simulink model "Stateflow_test"  (R2021a)
settings: Solver=FixedStepDiscrete  StartTime=0.0  StopTime=1000000  FixedStep=0.1  RelTol=1e-3
settings Model: EnablePacing=on  Creator=20201588  LastModifiedBy=20201588
settings DataIOCC: ExternalInput=k  SaveOutput=off  SignalLogging=off  DSMLogging=off  SaveTime=off  ReturnWorkspaceOutputs=off

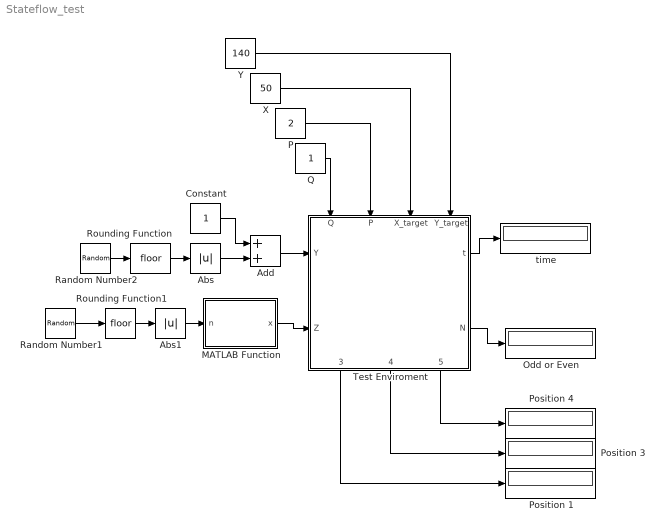
== system Stateflow_test ==
  Abs : Abs
  Abs1 : Abs
  Add : Sum
  Constant : Constant
  MATLAB Function : MATLAB Function  TreatAsAtomicUnit=on
  Odd or Even : Display
  P : Constant  Value=2
  Position 1 : Display
  Position 3 : Display
  Position 4 : Display
  Q : Constant
  Random Number1 : RandomNumber  Variance=100000  SampleTime=0.1
  Random Number2 : RandomNumber  Variance=100000  SampleTime=0.1
  Rounding Function : Rounding
  Rounding Function1 : Rounding
  Test Enviroment : Stateflow chart  TreatAsAtomicUnit=on
      settings: PortSchema="{\"entries\":[{\"content\":{\"sides\":[{\"content\":{\"connectorIds\":[\"In1\",\"In2\"]},\"type\":\"ConnectorPlacement.EquallySpacedRectSide\",\"uuid\":\"30c27bf2-aba7-402c-b200-cd809c499820\"},{\"content\":{\"connectorIds\":[\"Out1\",\"Out2\"],\"side\":\"RIGHT\"},\"type\":\"ConnectorPlacement.EquallySpacedRectSide\",\"uuid\":\"5fb1c3a1-970d-4595-8858-19f50385e32e\"},{\"content\":{\"connectorIds\":[\"In4\",\"In3\",\"In5\",\"In6\"],\"side\":\"TOP\"},\"type\":\"ConnectorPlacement.EquallySpacedRectSide\",\"uuid\":\"36195fad-53c8-499a-9c43-961bfbaf41e7\"},{\"content\":{\"connectorIds\":[\"Out3\",\"Out4\",\"Out5\"],\"side\":\"BOTTOM\"},\"type\":\"ConnectorPlacement.EquallySpacedRectSide\",\"uuid\":\"809a5c53-c969-4d66-b175-34124aee756d\"}]},\"type\":\"ConnectorPlacement.EquallySpacedConnector\",\"uuid\":\"2a5091d1-cc93-467a-a765-baae29c7acb5\"}],\"packageUris\":[\"http://schema.mathworks.com/mf0/Connector/R2020b\"],\"version\":\"1.0\"}"
  X : Constant  Value=50
  Y : Constant  Value=140
  time : Display
  wires:
  Test Enviroment/2(N) -> Odd or Even/1
  Random Number2/1 -> Rounding Function/1
  Test Enviroment/1(t) -> time/1
  Rounding Function/1 -> Abs/1
  MATLAB Function/1(x) -> Test Enviroment/2(Z)
  Rounding Function1/1 -> Abs1/1
  Abs1/1 -> MATLAB Function/1(n)
  Random Number1/1 -> Rounding Function1/1
  Abs/1 -> Add/2
  Add/1 -> Test Enviroment/1(Y)
  Constant/1 -> Add/1
  P/1 -> Test Enviroment/3(P)
  Q/1 -> Test Enviroment/4(Q)
  X/1 -> Test Enviroment/5(X_target)
  Y/1 -> Test Enviroment/6(Y_target)
  Test Enviroment/5(R_rad_target) -> Position 4/1
  Test Enviroment/4(X_rad_target) -> Position 3/1
  Test Enviroment/3(Z_rad_target) -> Position 1/1

== matlab function Stateflow_test/MATLAB Function ==
  data: n input; x output
function x = fcn(n)

r = randi([-10*n 10*n],n,n);

s = randi([1 n],1,1);
f = randi([1 n],1,1);

x = r(s,f);

== stateflow chart Stateflow_test/Test Enviroment ==
  state Odd_or_Even [parallel]
    settings: executionOrder=1
    state Sum_is_odd
      entry:
      X = 1; N = 0;
      during:
      X = rand(Y)+Z;
    state Sum_is_even
      entry:
      X = 2; N = 1;
      during:
      X = rand(Y)+Z;
    (default) -> Sum_is_odd
    Sum_is_odd -> Sum_is_even : [rem(X,2)==0]
    Sum_is_even -> Sum_is_odd : [rem(X,2)==1]
  state Time [parallel]
    settings: executionOrder=2
    state Time_1
      entry, during:
      p = rand(Y);
      t = elapsed(sec);
    state Time_2 [commented out]
      entry, during:
      T = elapsed(sec);
    (default) -> Time_1
    Time_2 -> Time_1 [commented out] : after(1,sec)
    Time_1 -> Time_2 [commented out] : after(1,sec)
  state Position_Example [parallel] [commented out]
    state Block_1 [parallel] [commented out]
      state Pick_Up_Block_1 [commented out]
        en, du:
        P1 =  0;
        exit:
        Pi_1 = 4;
      state Position_Block_1 [commented out]
        du, en:
        P1 = 5*elapsed(sec) + Pi_1;
      state Start [commented out]
        du,en:
        Pi_1 = 0;
      Position_Example.Block_1.Start -> Position_Block_1 [commented out]
      (default) -> Position_Example.Block_1.Start [commented out]
      Pick_Up_Block_1 -> Position_Block_1 [commented out] : [P == 0 & Q ==1 ]
      Position_Block_1 -> Pick_Up_Block_1 [commented out] : [P == 1 & Q == 1]
    state Block_2 [parallel] [commented out]
      state Pick_Up_Block_2 [commented out]
        en, du:
        P2 = 0;
        exit:
        Pi_2 = 4;
      state Position_Block_2 [commented out]
        du, en:
        P2 = 5*elapsed(sec) + Pi_2;
      state Start [commented out]
        du,en:
        Pi_2 = 0;
      Pick_Up_Block_2 -> Position_Block_2 [commented out] : [P == 0 & Q ==2 ]
      Position_Block_2 -> Pick_Up_Block_2 [commented out] : [P == 1 & Q == 2]
      Position_Example.Block_2.Start -> Position_Block_2 [commented out]
      (default) -> Position_Example.Block_2.Start [commented out]
  state Read_Table [parallel]
    settings: executionOrder=3
    state Lookup_Table
      en:
      X_start  =  -228;
      Y_start  = 79;
      [Red_X, Red_Z,  Red_R, ...
      Yel_X, Yel_Z, Yel_R, ...
      Tra_X, Tra_Z, Tra_R, step]  = Lookup;
    state Detecting_Stage
      %This is where the detection
      %of the block would happen
    state Moving_Stage_Yellow
      en,du:
      X_index = (X_target-X_start)/step;
      Y_index = (Y_target-Y_start)/step;
      X_rad_target = interp2(Yel_X,Y_index,X_index);
      R_rad_target = interp2(Yel_R,Y_index,X_index);
      Z_rad_target = interp2(Yel_Z,Y_index,X_index);
    state Moving_Stage_Red
      en,du:
      X_index = (X_target-X_start)/step;
      Y_index = (Y_target-Y_start)/step;
      X_rad_target = interp2(Red_X,Y_index,X_index);
      R_rad_target = interp2(Red_R,Y_index,X_index);
      Z_rad_target = interp2(Red_Z,Y_index,X_index);
    state Transport_Stage
      en,du:
      X_index = (X_target-X_start)/step;
      Y_index = (Y_target-Y_start)/step;
      X_rad_target = interp2(Tra_X,Y_index,X_index);
      R_rad_target = interp2(Tra_R,Y_index,X_index);
      Z_rad_target = interp2(Tra_Z,Y_index,X_index);
    (default) -> Lookup_Table
    Lookup_Table -> Detecting_Stage
    Detecting_Stage -> Moving_Stage_Yellow [order 2] : [Q == 2 & P ==1]
    Detecting_Stage -> Moving_Stage_Red [order 1] : [Q == 1 & P ==1]
    Moving_Stage_Red -> Transport_Stage : [P == 2]
    Moving_Stage_Yellow -> Transport_Stage : [P == 2]
  data: n function_input; x function_output; P1 function_output; P2 function_output; P3 function_output; P4 function_output; P5 function_output; P6 function_output; P7 function_output; P8 function_output; P9 function_output; step_size function_output; Y input; Z input; X local; t output; N output; p local; P input; Q input; Pi_2 local; Pi_1 local; Red_R local; Red_Z local; Red_X local; Tra_X local; Yel_R local; Yel_X local; Yel_Z local; Tra_Z local; step local; Y_start local; X_start local; Z_rad_target output; X_rad_target output; R_rad_target output; X_target input; Y_target input; Tra_R local; X_index local; Y_index local
  function x = rand(n):
    | function x = rand(n)
    |  
    | r = randi([-10*n 10*n],n,n);
    | 
    | s = randi([1 n],1,1);
    | f = randi([1 n],1,1);
    | 
    | x = r(s,f);
  function [P1, P2, P3, P4, P5,  P6,  P7,  P8,  P9, step_size]= Lookup:
    | function [P1, P2, P3, P4, P5,  P6,  P7,  P8,  P9, step_size]= Lookup
    | 
    | step_size = 20
    | 
    | P1 = ...
    |   [0.078490748900463925 0 0 0 0 0 0;
    |    -0.14160324448913111 -0.049572307843604724 0.12708300072520992 0 0 0 ...
    |    0;
    |    -0.27157787377661163 -0.20182258283986637 -0.10634227096077699 0.048525204061919937 ...
    |    0 0 0;
    |    -0.37215450602130229 -0.30994030328141381 -0.23070086145651506 -0.12513068019242732 ...
    |    0.044207338161135111 0 0;
    |    -0.45597476566310996 -0.39644723094061213 -0.32358159546482551 -0.23266896174672444 ...
    |    -0.11132586814638003 0.10678216745830364 0;
    |    -0.52822091878882982 -0.46869829447830874 -0.39813136114620756 -0.3135156344249258 ...
    |    -0.20797697259670342 -0.061121896669658671 0;
    |    -0.59138527368032068 -0.52990747874252764 -0.45929417119146188 -0.37726504619144469 ...
    |    -0.27901154079820384 -0.15302076809051285 0.0499859200990351;
    |    -0.64643227421234584 -0.58139905329097474 -0.5091959536765388 -0.42771137003577658 ...
    |    -0.33297424363263062 -0.21676008945412273 -0.054434792366532522;
    |    -0.62328641003273344 -0.54856621140117323 -0.46648547704422505 -0.3732914885966841 ...
    |    -0.26219124059014348 -0.1162498375777507 0;
    |    -0.65477765533194343 -0.57731612637156482 -0.49417897981862507 -0.40149598471752612 ...
    |    -0.29308567320354412 -0.15527223637806487 0;
    |    -0.67454045864903067 -0.59493539199982293 -0.510868815105908 -0.41825451853521306 ...
    |    -0.31113343840230134 -0.17725387432785519 0;
    |    -0.6008842036628036 -0.51645247029269337 -0.42382031113568408 -0.3170789405401413 ...
    |    -0.18438303533059774 0 0;
    |    -0.67454045864903067 -0.59493539199982293 -0.510868815105908 -0.41825451853521306 ...
    |    -0.31113343840230134 -0.17725387432785519 0;
    |    -0.65477765533194343 -0.57731612637156482 -0.49417897981862507 -0.40149598471752612 ...
    |    -0.29308567320354412 -0.15527223637806487 0;
    |    -0.62328641003273344 -0.54856621140117323 -0.46648547704422505 -0.3732914885966841 ...
    |    -0.26219124059014348 -0.1162498375777507 0;
    |    -0.64643227421234584 -0.58139905329097474 -0.5091959536765388 -0.42771137003577658 ...
    |    -0.33297424363263062 -0.21676008945412273 -0.054434792366532522;
    |    -0.59138527368032068 -0.52990747874252764 -0.45929417119146188 -0.37726504619144469 ...
    |    -0.27901154079820384 -0.15302076809051285 0.0499859200990351;
    |    -0.52822091878882982 -0.46869829447830874 -0.39813136114620756 -0.3135156344249258 ...
    |    -0.20797697259670342 -0.061121896669658671 0;
    |    -0.45597476566310996 -0.39644723094061213 -0.32358159546482551 -0.23266896174672444 ...
    |    -0.11132586814638003 0.10678216745830364 0;
    |    -0.37215450602130229 -0.30994030328141381 -0.23070086145651506 -0.12513068019242732 ...
    |    0.044207338161135111 0 0;
    |    -0.27157787377661163 -0.20182258283986637 -0.10634227096077699 0.048525204061919937 ...
    |    0 0 0;
    |    -0.14160324448913111 -0.049572307843604724 0.12708300072520992 0 0 0 ...
    |    0;
    |    0.078490748900463925 0 0 0 0 0 0];
    | P2 = ...
    |   [-0.12914851440826922 0 0 0 0 0 0;
    |    -0.031147893091569411 -0.077606350910947919 -0.14238184107600749 0 0 ...
    |    0 0;
    |    0.038115006213386052 0.00097753000030033452 -0.049502944336502347 -0.11903370925601538 ...
    |    0 0 0;
    |    0.088172973459990187 0.057915795871910543 0.016451058436103165 -0.039786051111986041 ...
    |    -0.11746414751217649 0 0;
    |    0.12320986517913864 0.099126747790600628 0.064776879140110641 0.017502499912164002 ...
    |    -0.046941591530162037 -0.13735685373267448 0;
    |    0.1455634435709153 0.12775542375045904 0.099864536107933291 0.059724492124420374 ...
    |    0.0042794148117395675 -0.072074838684885761 0;
    |    0.15698816571742835 0.14597603798865905 0.12441834465360993 0.090523742090328235 ...
    |    0.042001398835270945 -0.02510904800516426 -0.11955852667623298;
    |    0.15935403780028756 0.15576457968830729 0.14053907023566314 0.11231467916400005 ...
    |    0.069434622529717827 0.0089891923775578877 -0.075290820322378632;
    |    0.15929172088395394 0.15016609924800148 0.12698191064896727 0.0886980038252953 ...
    |    0.033179981423454109 -0.044399102796648091 0;
    |    0.15903111902237949 0.15519807407823663 0.13611481885448781 0.10132963703365482 ...
    |    0.049298666564871779 -0.023914081850700819 0;
    |    0.15751883351380158 0.15736682441418084 0.14100746879651566 0.10844319967004758 ...
    |    0.058520174583554761 -0.012192524522075769 0;
    |    0.1579339306852009 0.14253431690789742 0.11073471576986624 0.061519876623784726 ...
    |    -0.0083753026802587047 0 0;
    |    0.15751883351380158 0.15736682441418084 0.14100746879651566 0.10844319967004758 ...
    |    0.058520174583554761 -0.012192524522075769 0;
    |    0.15903111902237949 0.15519807407823663 0.13611481885448781 0.10132963703365482 ...
    |    0.049298666564871779 -0.023914081850700819 0;
    |    0.15929172088395394 0.15016609924800148 0.12698191064896727 0.0886980038252953 ...
    |    0.033179981423454109 -0.044399102796648091 0;
    |    0.15935403780028756 0.15576457968830729 0.14053907023566314 0.11231467916400005 ...
    |    0.069434622529717827 0.0089891923775578877 -0.075290820322378632;
    |    0.15698816571742835 0.14597603798865905 0.12441834465360993 0.090523742090328235 ...
    |    0.042001398835270945 -0.02510904800516426 -0.11955852667623298;
    |    0.1455634435709153 0.12775542375045904 0.099864536107933291 0.059724492124420374 ...
    |    0.0042794148117395675 -0.072074838684885761 0;
    |    0.12320986517913864 0.099126747790600628 0.064776879140110641 0.017502499912164002 ...
    |    -0.046941591530162037 -0.13735685373267448 0;
    |    0.088172973459990187 0.057915795871910543 0.016451058436103165 -0.039786051111986041 ...
    |    -0.11746414751217649 0 0;
    |    0.038115006213386052 0.00097753000030033452 -0.049502944336502347 -0.11903370925601538 ...
    |    0 0 0;
    |    -0.031147893091569411 -0.077606350910947919 -0.14238184107600749 0 0 ...
    |    0 0;
    |    -0.12914851440826922 0 0 0 0 0 0];
    | P3 = ...
    |   [-1.1555280696863055 0 0 0 0 0 0;
    |    -1.1192205659593462 -1.0414792570758407 -0.97020857536930272 0 0 0 0 ...
    |    ;
    |    -1.076523722378983 -0.99442110620371293 -0.92022194958143655 -0.85354174926493276 ...
    |    0 0 0;
    |    -1.025793907189114 -0.939403607044929 -0.86268498768041613 -0.79486160328000632 ...
    |    -0.73499578368810314 0 0;
    |    -0.9648803301212161 -0.87465454274782362 -0.7962280648859561 -0.72822149452105855 ...
    |    -0.66920466660723954 -0.617844488214677 0;
    |    -0.89099469902914064 -0.79805571523150021 -0.71934652850130743 -0.65261016858449106 ...
    |    -0.59578454762305888 -0.5471108502163885 0;
    |    -0.80062541277456556 -0.70721682979106137 -0.63053013816735171 -0.5671412488145694 ...
    |    -0.51426512799322155 -0.46972040884091021 -0.43182315125830661;
    |    -0.68964667050168171 -0.59974374696942356 -0.52852816890339194 -0.4712616750560702 ...
    |    -0.42449711714228811 -0.38574650382157327 -0.35320392615379503;
    |    -0.4738513364947603 -0.412793289970719 -0.36503799768109646 -0.32682665292994068 ...
    |    -0.29564281653907476 -0.26975807296212945 0;
    |    -0.32942303811214763 -0.28407437825928533 -0.2494696508978248 -0.22225530228522308 ...
    |    -0.20032238076082171 -0.18228559876685382 0;
    |    -0.16930377815578745 -0.14496139639150155 -0.12670608739343886 -0.11251710743602975 ...
    |    -0.10117618903756062 -0.09190625132479012 0;
    |    0 0 0 0 0 0 0;
    |    0.16930377815578745 0.14496139639150155 0.12670608739343886 0.11251710743602975 ...
    |    0.10117618903756062 0.09190625132479012 0;
    |    0.32942303811214763 0.28407437825928533 0.2494696508978248 0.22225530228522308 ...
    |    0.20032238076082171 0.18228559876685382 0;
    |    0.4738513364947603 0.412793289970719 0.36503799768109646 0.32682665292994068 ...
    |    0.29564281653907476 0.26975807296212945 0;
    |    0.68964667050168171 0.59974374696942356 0.52852816890339194 0.4712616750560702 ...
    |    0.42449711714228811 0.38574650382157327 0.35320392615379503;
    |    0.80062541277456556 0.70721682979106137 0.63053013816735171 0.5671412488145694 ...
    |    0.51426512799322155 0.46972040884091021 0.43182315125830661;
    |    0.89099469902914064 0.79805571523150021 0.71934652850130743 0.65261016858449106 ...
    |    0.59578454762305888 0.5471108502163885 0;
    |    0.9648803301212161 0.87465454274782362 0.7962280648859561 0.72822149452105855 ...
    |    0.66920466660723954 0.617844488214677 0;
    |    1.025793907189114 0.939403607044929 0.86268498768041613 0.79486160328000632 ...
    |    0.73499578368810314 0 0;
    |    1.076523722378983 0.99442110620371293 0.92022194958143655 0.85354174926493276 ...
    |    0 0 0;
    |    1.1192205659593462 1.0414792570758407 0.97020857536930272 0 0 0 0;
    |    1.1555280696863055 0 0 0 0 0 0];
    | P4 = ...
    |   [-0.11480438890444414 -0.0087043704871341727 0 0 0 0 0;
    |    -0.27129154221375518 -0.19669467676343674 -0.093513525421083779 0.084162799376508335 ...
    |    0 0 0;
    |    -0.38979410217880406 -0.32466498232115132 -0.24156701330429597 -0.13095572032037739 ...
    |    0.044976045332462418 0 0;
    |    -0.48861664005099803 -0.42686197626553057 -0.35124331883001292 -0.25724872369268215 ...
    |    -0.13345504395339669 0.072723448912593427 0;
    |    -0.57476980602955541 -0.51324504399375992 -0.44023460899805017 -0.35307531411572796 ...
    |    -0.24569010559136686 -0.10162396951576309 0;
    |    -0.65167507358591581 -0.58813506580271135 -0.51496283941836685 -0.43035746187103235 ...
    |    -0.33028026714588782 -0.20548593687598274 -0.025768105024669096;
    |    -0.72098091250864249 -0.65350015115864957 -0.57824932702273313 -0.49377438215542246 ...
    |    -0.39691262889478879 -0.28117521366138309 -0.13011965407856094;
    |    -0.7830172500349053 -0.70989177107989809 -0.63118257048769255 -0.54535151914097724 ...
    |    -0.44949827412252308 -0.33834070215201667 -0.20037307019867423;
    |    -0.7567437924386452 -0.67378365591319223 -0.58580519618607074 -0.48976303757431194 ...
    |    -0.38085139229755555 -0.249790070573472 0;
    |    -0.792557865764006 -0.70537233505681729 -0.61512953492812483 -0.51839872984958613 ...
    |    -0.41047590879780493 -0.28313810581564314 0;
    |    -0.81529405574172442 -0.72493523237816626 -0.6329775035109414 -0.53559153202907717 ...
    |    -0.42802771488078972 -0.30253084067127051 0;
    |    -0.82312145765711964 -0.73157564397637886 -0.63897831058807675 -0.541330671486956 ...
    |    -0.433847885204258 -0.30890560112112947 0;
    |    -0.81529405574172442 -0.72493523237816626 -0.6329775035109414 -0.53559153202907717 ...
    |    -0.42802771488078972 -0.30253084067127051 0;
    |    -0.792557865764006 -0.70537233505681729 -0.61512953492812483 -0.51839872984958613 ...
    |    -0.41047590879780493 -0.28313810581564314 0;
    |    -0.7567437924386452 -0.67378365591319223 -0.58580519618607074 -0.48976303757431194 ...
    |    -0.38085139229755555 -0.249790070573472 0;
    |    -0.7830172500349053 -0.70989177107989809 -0.63118257048769255 -0.54535151914097724 ...
    |    -0.44949827412252308 -0.33834070215201667 -0.20037307019867423;
    |    -0.72098091250864249 -0.65350015115864957 -0.57824932702273313 -0.49377438215542246 ...
    |    -0.39691262889478879 -0.28117521366138309 -0.13011965407856094;
    |    -0.65167507358591581 -0.58813506580271135 -0.51496283941836685 -0.43035746187103235 ...
    |    -0.33028026714588782 -0.20548593687598274 -0.025768105024669096;
    |    -0.57476980602955541 -0.51324504399375992 -0.44023460899805017 -0.35307531411572796 ...
    |    -0.24569010559136686 -0.10162396951576309 0;
    |    -0.48861664005099803 -0.42686197626553057 -0.35124331883001292 -0.25724872369268215 ...
    |    -0.13345504395339669 0.072723448912593427 0;
    |    -0.38979410217880406 -0.32466498232115132 -0.24156701330429597 -0.13095572032037739 ...
    |    0.044976045332462418 0 0;
    |    -0.27129154221375518 -0.19669467676343674 -0.093513525421083779 0.084162799376508335 ...
    |    0 0 0;
    |    -0.11480438890444414 -0.0087043704871341727 0 0 0 0 0];
    | P5 = ...
    |   [-0.24673541637606086 -0.32708140148903825 0 0 0 0 0;
    |    -0.13508527788696956 -0.1867808782122489 -0.26272322297635359 -0.39310787333689307 ...
    |    0 0 0;
    |    -0.060953659048357721 -0.10031444194936018 -0.1552909799718652 -0.23470001769543178 ...
    |    -0.36685148097996906 0 0;
    |    -0.0092113129716279319 -0.040306717724784467 -0.083811266736301737 -0.14456147945646064 ...
    |    -0.23284565228895937 -0.385899385174958 0;
    |    0.026017251538530208 0.0019019004603818112 -0.033206661496261718 -0.082695304528894634 ...
    |    -0.15245530540477917 -0.2566180159405671 0;
    |    0.047834799469926408 0.030509609781595372 0.0026474446463063688 -0.038432301700045822 ...
    |    -0.096780079170587188 -0.18052517996638445 -0.31413735810011628;
    |    0.058440614251111307 0.048228861120119912 0.027213744691138853 -0.0068195006255562891 ...
    |    -0.056882886702900044 -0.12849380440497765 -0.23532083433036152;
    |    0.059997925447379551 0.057359742052474995 0.04300268328167365 0.015167128181215208 ...
    |    -0.028402757182387665 -0.091750773249466525 -0.18415855458984426;
    |    0.060274717385612374 0.05219950591946846 0.029746745607967834 -0.0086767999410887 ...
    |    -0.066135754029155072 -0.14964580186696502 0;
    |    0.0595561004637293 0.056850570603744856 0.038706352886425155 0.0041267885277485638 ...
    |    -0.049263580272588724 -0.12719263893476587 0;
    |    0.057774756129627167 0.058767823535331887 0.043455477373128604 0.011286879739403052 ...
    |    -0.039680162380876953 -0.11448297026704295 0;
    |    0.056926059656801822 0.059248057442413016 0.044928372112162267 0.013585053051782432 ...
    |    -0.036573606009370083 -0.11036444284949966 0;
    |    0.057774756129627167 0.058767823535331887 0.043455477373128604 0.011286879739403052 ...
    |    -0.039680162380876953 -0.11448297026704295 0;
    |    0.0595561004637293 0.056850570603744856 0.038706352886425155 0.0041267885277485638 ...
    |    -0.049263580272588724 -0.12719263893476587 0;
    |    0.060274717385612374 0.05219950591946846 0.029746745607967834 -0.0086767999410887 ...
    |    -0.066135754029155072 -0.14964580186696502 0;
    |    0.059997925447379551 0.057359742052474995 0.04300268328167365 0.015167128181215208 ...
    |    -0.028402757182387665 -0.091750773249466525 -0.18415855458984426;
    |    0.058440614251111307 0.048228861120119912 0.027213744691138853 -0.0068195006255562891 ...
    |    -0.056882886702900044 -0.12849380440497765 -0.23532083433036152;
    |    0.047834799469926408 0.030509609781595372 0.0026474446463063688 -0.038432301700045822 ...
    |    -0.096780079170587188 -0.18052517996638445 -0.31413735810011628;
    |    0.026017251538530208 0.0019019004603818112 -0.033206661496261718 -0.082695304528894634 ...
    |    -0.15245530540477917 -0.2566180159405671 0;
    |    -0.0092113129716279319 -0.040306717724784467 -0.083811266736301737 -0.14456147945646064 ...
    |    -0.23284565228895937 -0.385899385174958 0;
    |    -0.060953659048357721 -0.10031444194936018 -0.1552909799718652 -0.23470001769543178 ...
    |    -0.36685148097996906 0 0;
    |    -0.13508527788696956 -0.1867808782122489 -0.26272322297635359 -0.39310787333689307 ...
    |    0 0 0;
    |    -0.24673541637606086 -0.32708140148903825 0 0 0 0 0];
    | P6 = ...
    |   [-1.1555280696863055 -1.0820193588220757 0 0 0 0 0;
    |    -1.1192205659593462 -1.0414792570758407 -0.97020857536930272 -0.90526888306939379 ...
    |    0 0 0;
    |    -1.076523722378983 -0.99442110620371293 -0.92022194958143655 -0.85354174926493276 ...
    |    -0.79380132694509531 0 0;
    |    -1.025793907189114 -0.939403607044929 -0.86268498768041613 -0.79486160328000632 ...
    |    -0.73499578368810314 -0.68212542337860449 0;
    |    -0.9648803301212161 -0.87465454274782362 -0.7962280648859561 -0.72822149452105855 ...
    |    -0.66920466660723954 -0.617844488214677 0;
    |    -0.89099469902914064 -0.79805571523150021 -0.71934652850130743 -0.65261016858449106 ...
    |    -0.59578454762305888 -0.5471108502163885 -0.50514002667699287;
    |    -0.80062541277456556 -0.70721682979106137 -0.63053013816735171 -0.5671412488145694 ...
    |    -0.51426512799322155 -0.46972040884091021 -0.43182315125830661;
    |    -0.68964667050168171 -0.59974374696942356 -0.52852816890339194 -0.4712616750560702 ...
    |    -0.42449711714228811 -0.38574650382157327 -0.35320392615379503;
    |    -0.4738513364947603 -0.412793289970719 -0.36503799768109646 -0.32682665292994068 ...
    |    -0.29564281653907476 -0.26975807296212945 0;
    |    -0.32942303811214763 -0.28407437825928533 -0.2494696508978248 -0.22225530228522308 ...
    |    -0.20032238076082171 -0.18228559876685382 0;
    |    -0.16930377815578745 -0.14496139639150155 -0.12670608739343886 -0.11251710743602975 ...
    |    -0.10117618903756062 -0.09190625132479012 0;
    |    0 0 0 0 0 0 0;
    |    0.16930377815578745 0.14496139639150155 0.12670608739343886 0.11251710743602975 ...
    |    0.10117618903756062 0.09190625132479012 0;
    |    0.32942303811214763 0.28407437825928533 0.2494696508978248 0.22225530228522308 ...
    |    0.20032238076082171 0.18228559876685382 0;
    |    0.4738513364947603 0.412793289970719 0.36503799768109646 0.32682665292994068 ...
    |    0.29564281653907476 0.26975807296212945 0;
    |    0.68964667050168171 0.59974374696942356 0.52852816890339194 0.4712616750560702 ...
    |    0.42449711714228811 0.38574650382157327 0.35320392615379503;
    |    0.80062541277456556 0.70721682979106137 0.63053013816735171 0.5671412488145694 ...
    |    0.51426512799322155 0.46972040884091021 0.43182315125830661;
    |    0.89099469902914064 0.79805571523150021 0.71934652850130743 0.65261016858449106 ...
    |    0.59578454762305888 0.5471108502163885 0.50514002667699287;
    |    0.9648803301212161 0.87465454274782362 0.7962280648859561 0.72822149452105855 ...
    |    0.66920466660723954 0.617844488214677 0;
    |    1.025793907189114 0.939403607044929 0.86268498768041613 0.79486160328000632 ...
    |    0.73499578368810314 0.68212542337860449 0;
    |    1.076523722378983 0.99442110620371293 0.92022194958143655 0.85354174926493276 ...
    |    0.79380132694509531 0 0;
    |    1.1192205659593462 1.0414792570758407 0.97020857536930272 0.90526888306939379 ...
    |    0 0 0;
    |    1.1555280696863055 1.0820193588220757 0 0 0 0 0];
    | P7 = ...
    |   [0 0 0 0 0 0;
    |    0 0 0 0 0 0;
    |    0.26997556673912604 0 0 0 0 0;
    |    0.11743620156601944 0.20307050439264948 0.37122632241072184 0 0 0;
    |    0.02602560457586605 0.088691261935096743 0.18242876750271442 0.364819492114137 ...
    |    0 0;
    |    -0.038165732644201034 0.013852535702424071 0.086774306707618459 0.19753391630095496 ...
    |    0.52091363996896567 0;
    |    -1.2050148353955614 -0.039528025759173989 0.022811680620281695 0.11121081654844342 ...
    |    0.25569902811592049 0;
    |    -0.12016969837912329 -1.1942629572053136 -0.022384361516127989 0.054536264394245346 ...
    |    0.16891547584301525 0.42873811693533664;
    |    -0.14564410050636142 -0.10616507435082738 -0.054209197726544506 0.015941432729109396 ...
    |    0.11604250793680168 0.2892538075728463;
    |    -0.16332874068700814 -0.12499203752417062 -1.1897083201679897 -0.0093776875143855767 ...
    |    0.082972146915499922 0.23057545613413558;
    |    -0.17391638828449343 -0.13595108131413222 -0.087698389556319409 -0.023802892974453073 ...
    |    0.064559922063085473 0.20121230366815185;
    |    -0.17746956647501461 -0.1395576386441334 -0.091696248105389608 -0.02849422391601486 ...
    |    0.058629730672907825 0.1921079523514149;
    |    -0.17391638828449343 -0.13595108131413222 -0.087698389556319409 -0.023802892974453073 ...
    |    0.064559922063085473 0.20121230366815185;
    |    -0.16332874068700814 -0.12499203752417062 -1.1897083201679897 -0.0093776875143855767 ...
    |    0.082972146915499922 0.23057545613413558;
    |    -0.14564410050636142 -0.10616507435082738 -0.054209197726544506 0.015941432729109396 ...
    |    0.11604250793680168 0.2892538075728463;
    |    -0.12016969837912329 -1.1942629572053136 -0.022384361516127989 0.054536264394245346 ...
    |    0.16891547584301525 0.42873811693533664;
    |    -1.2050148353955614 -0.039528025759173989 0.022811680620281695 0.11121081654844342 ...
    |    0.25569902811592049 0;
    |    -0.038165732644201034 0.013852535702424071 0.086774306707618459 0.19753391630095496 ...
    |    0.52091363996896567 0;
    |    0.02602560457586605 0.088691261935096743 0.18242876750271442 0.364819492114137 ...
    |    0 0;
    |    0.11743620156601944 0.20307050439264948 0.37122632241072184 0 0 0;
    |    0.26997556673912604 0 0 0 0 0];
    | P8 = ...
    |   [0 0 0 0 0 0;
    |    0 0 0 0 0 0;
    |    0.38509141474537723 0 0 0 0 0;
    |    0.44057985856937665 0.40631221377665971 0.36275327638414057 0 0 0;
    |    0.48448139805888069 0.45369079009690211 0.41386901461354614 0.36381807721266984 ...
    |    0 0;
    |    0.51760517821625829 0.49072016649521988 0.45459059107985883 0.408293437295171 ...
    |    0.350562193258226 0;
    |    -1.9291450306000577 0.51830127084204136 0.48612292565974546 0.443356555045519 ...
    |    0.38919214616911008 0;
    |    0.55386389919269408 -1.9091006280564233 0.50947956401061334 0.47015029270233877 ...
    |    0.41906515293861196 0.35525037094710482;
    |    0.55914344134010718 0.54910103180000092 0.525716369905997 0.48964572099879528 ...
    |    0.44119836684871055 0.37992668569633564;
    |    0.55881865225642435 0.55524782538883444 -1.90098142506241 0.50273748985438682 ...
    |    0.45638421609582747 0.39697477121414376;
    |    0.556345552393312 0.55777682644656323 0.54155625336518487 0.5102133817995631 ...
    |    0.46523037625857577 0.40697339476621164;
    |    0.55504827959824254 0.55839163647462342 0.543285517193445 0.51263641508894264 ...
    |    0.4681327747611117 0.41026769400401464;
    |    0.556345552393312 0.55777682644656323 0.54155625336518487 0.5102133817995631 ...
    |    0.46523037625857577 0.40697339476621164;
    |    0.55881865225642435 0.55524782538883444 -1.90098142506241 0.50273748985438682 ...
    |    0.45638421609582747 0.39697477121414376;
    |    0.55914344134010718 0.54910103180000092 0.525716369905997 0.48964572099879528 ...
    |    0.44119836684871055 0.37992668569633564;
    |    0.55386389919269408 -1.9091006280564233 0.50947956401061334 0.47015029270233877 ...
    |    0.41906515293861196 0.35525037094710482;
    |    -1.9291450306000577 0.51830127084204136 0.48612292565974546 0.443356555045519 ...
    |    0.38919214616911008 0;
    |    0.51760517821625829 0.49072016649521988 0.45459059107985883 0.408293437295171 ...
    |    0.350562193258226 0;
    |    0.48448139805888069 0.45369079009690211 0.41386901461354614 0.36381807721266984 ...
    |    0 0;
    |    0.44057985856937665 0.40631221377665971 0.36275327638414057 0 0 0;
    |    0.38509141474537723 0 0 0 0 0];
    | P9 = ...
    |   [0 0 0 0 0 0;
    |    0 0 0 0 0 0;
    |    -1.076523722378983 0 0 0 0 0;
    |    -1.025793907189114 -0.939403607044929 -0.86268498768041613 0 0 0;
    |    -0.9648803301212161 -0.87465454274782362 -0.7962280648859561 -0.72822149452105855 ...
    |    0 0;
    |    -0.89099469902914064 -0.79805571523150021 -0.71934652850130743 -0.65261016858449106 ...
    |    -0.59578454762305888 0;
    |    -0.80062541277456556 -0.70721682979106137 -0.63053013816735171 -0.5671412488145694 ...
    |    -0.51426512799322155 0;
    |    -0.68964667050168171 -0.59974374696942356 -0.52852816890339194 -0.4712616750560702 ...
    |    -0.42449711714228811 -0.38574650382157327;
    |    -0.55395250864102774 -0.4738513364947603 -0.412793289970719 -0.36503799768109646 ...
    |    -0.32682665292994068 -0.29564281653907476;
    |    -0.39112544696902912 -0.32942303811214763 -0.28407437825928533 -0.2494696508978248 ...
    |    -0.22225530228522308 -0.20032238076082171;
    |    -0.20333608402827572 -0.16930377815578745 -0.14496139639150155 -0.12670608739343886 ...
    |    -0.11251710743602975 -0.10117618903756062;
    |    0 0 0 0 0 0;
    |    0.20333608402827572 0.16930377815578745 0.14496139639150155 0.12670608739343886 ...
    |    0.11251710743602975 0.10117618903756062;
    |    0.39112544696902912 0.32942303811214763 0.28407437825928533 0.2494696508978248 ...
    |    0.22225530228522308 0.20032238076082171;
    |    0.55395250864102774 0.4738513364947603 0.412793289970719 0.36503799768109646 ...
    |    0.32682665292994068 0.29564281653907476;
    |    0.68964667050168171 0.59974374696942356 0.52852816890339194 0.4712616750560702 ...
    |    0.42449711714228811 0.38574650382157327;
    |    0.80062541277456556 0.70721682979106137 0.63053013816735171 0.5671412488145694 ...
    |    0.51426512799322155 0;
    |    0.89099469902914064 0.79805571523150021 0.71934652850130743 0.65261016858449106 ...
    |    0.59578454762305888 0;
    |    0.9648803301212161 0.87465454274782362 0.7962280648859561 0.72822149452105855 ...
    |    0 0;
    |    1.025793907189114 0.939403607044929 0.86268498768041613 0 0 0;
    |    1.076523722378983 0 0 0 0 0];
